simulink model "Simulink_TEP"  (R2024a)
settings: Solver=FixedStepAuto  StartTime=0.0  StopTime=5  FixedStep=1/3600  RelTol=1e-3
model workspace (MAT data in the model file):
  AD : Simulink.Parameter (value not decoded)
  AG : Simulink.Parameter (value not decoded)
  AH : Simulink.Parameter (value not decoded)
  AV : Simulink.Parameter (value not decoded)
  AVP : Simulink.Parameter (value not decoded)
  BCHL : Simulink.Parameter (value not decoded)
  BCHV : Simulink.Parameter (value not decoded)
  BD : Simulink.Parameter (value not decoded)
  BG : Simulink.Parameter (value not decoded)
  BH : Simulink.Parameter (value not decoded)
  BVP : Simulink.Parameter (value not decoded)
  CD : Simulink.Parameter (value not decoded)
  CG : Simulink.Parameter (value not decoded)
  CH : Simulink.Parameter (value not decoded)
  CVP : Simulink.Parameter (value not decoded)
  XMW : Simulink.Parameter (value not decoded)
symbols that are objects in the model workspace (value not decoded): AD, AG, AH, AV, AVP, BD, BG, BH, BVP, CD, CG, CH, CVP, XMW
undefined symbols (not defined in the file or in its folder): magnitude, SETPT, XMEAS, XMV
libraries: mylib x165, dspindex x17
(part 2 of 10)

== system Simulink_TEP/D Feed Stream 4/HST(4) Molar Enthalpy of Stream 4 MBtu//lb-mol ==
  TST(4) : Inport
  XST(I,4) : Inport  Port=2
  "Enthalpy of Stream " : mylib/Enthalpy of Stream   SystemSampleTime=-1  VariantActivationTime=update diagram  AllowFlexibleInterface=on  Latency=0  AutoFrameSizeCalculation=off
  ITY : Constant
  HST(4) : Outport  VectorParamsAs1DForOutWhenUnconnected=off
  wires:
  ITY/1 -> "Enthalpy of Stream "/1
  TST(4)/1 -> "Enthalpy of Stream "/2
  XST(I,4)/1 -> "Enthalpy of Stream "/3
  "Enthalpy of Stream "/1 -> HST(4)/1

== system Simulink_TEP/D Feed Stream 4/XST(I;4) Composition of Stream 4  ==
  TESUB8(1) : Inport
  TESUB8(2) : Inport  Port=2
  IDV(1) : Inport  Port=3
  IDV(2) : Inport  Port=4
  Bus Creator : BusCreator  Inputs=4
  Bus to Vector : BusToVector
  Constant : Constant  Value=0.03
  Constant1 : Constant  Value=2.43719e-3
  Constant2 : Constant  Value=0.005
  Constant3 : Constant
  Constant4 : Constant  Value=[XST4_D;XST4_E;XST4_F;XST4_G;XST4_H]
  Product : Product
  Product1 : Product
  Product2 : Product
  XST(1,4) : Sum  Inputs=+--
  XST(2,4) : Sum
  XST(3,4) : Sum  Inputs=+--
  XST(I;4) : Outport  PortDimensions=8  VectorParamsAs1DForOutWhenUnconnected=off
  wires:
  TESUB8(1)/1 -> XST(1,4)/1
  XST(1,4)/1 -> Bus Creator/1, XST(3,4)/2
  Product1/1 -> XST(1,4)/3
  IDV(1)/1 -> Product/1
  Constant3/1 -> XST(3,4)/1
  Product/1 -> XST(1,4)/2
  XST(2,4)/1 -> Bus Creator/2, XST(3,4)/3
  IDV(2)/1 -> Product2/1, Product1/1
  Constant2/1 -> Product2/2
  Constant/1 -> Product/2
  Constant1/1 -> Product1/2
  TESUB8(2)/1 -> XST(2,4)/1
  Product2/1 -> XST(2,4)/2
  XST(3,4)/1 -> Bus Creator/3
  Constant4/1 -> Bus Creator/4
  Bus Creator/1 -> Bus to Vector/1
  Bus to Vector/1 -> XST(I;4)/1

== system Simulink_TEP/Disturbances/Subsystem1 ==
  IDVWLK(2) : Inport
  Bus Creator : BusCreator  Inputs=6
  Bus Selector : BusSelector  OutputSignals=ADIST,BDIST,CDIST,DDIST,TNEXT,TLAST
  Delay{,1..5} (6 alike) : Delay  DelayLength=1  InitialCondition=0
  Subsystem2 : Subsystem
  TESUB8 : mylib/TESUB8  SystemSampleTime=-1  VariantActivationTime=update diagram  AllowFlexibleInterface=on  Latency=0  AutoFrameSizeCalculation=off
  TESUB8(2,Time) : Outport  PortDimensions=1  VectorParamsAs1DForOutWhenUnconnected=off
  tag scope: DIST2=global
  wires:
  TESUB8/1 -> TESUB8(2,Time)/1
  Bus Selector/6 -> Delay5/1  "<TLAST>"
  Bus Selector/5 -> Delay4/1  "<TNEXT>"
  Delay1/1 -> Bus Creator/2  "BDIST"
  Delay4/1 -> Bus Creator/5  "TNEXT"
  Delay5/1 -> Bus Creator/6  "TLAST"
  Subsystem2/1(DIST_NEW) -> TESUB8/1, Bus Selector/1
  IDVWLK(2)/1 -> Subsystem2/1(IDVWLK)
  Delay3/1 -> Bus Creator/4  "DDIST"
  Bus Selector/3 -> Delay2/1  "<CDIST>"
  Bus Selector/2 -> Delay1/1  "<BDIST>"
  Bus Creator/1 -> [DIST2], Subsystem2/2(DIST)
  Bus Selector/1 -> Delay/1  "<ADIST>"
  Delay2/1 -> Bus Creator/3  "CDIST"
  Bus Selector/4 -> Delay3/1  "<DDIST>"
  Delay/1 -> Bus Creator/1  "ADIST"

== system Simulink_TEP/Disturbances/Subsystem10 ==
  IDVWLK(10) : Inport
  Bus Creator : BusCreator  Inputs=6
  Bus Selector : BusSelector  OutputSignals=ADIST,BDIST,CDIST,DDIST,TNEXT,TLAST
  Delay{,1..6} (7 alike) : Delay  DelayLength=1  InitialCondition=0
  Subsystem3 : Subsystem
  TESUB8 : mylib/TESUB8  SystemSampleTime=-1  VariantActivationTime=update diagram  AllowFlexibleInterface=on  Latency=0  AutoFrameSizeCalculation=off
  TESUB8(10,Time) : Outport  VectorParamsAs1DForOutWhenUnconnected=off
  tag scope: DIST10=global, SWLK_10=global
  wires:
  TESUB8/1 -> TESUB8(10,Time)/1
  Delay/1 -> Bus Creator/1  "ADIST"
  Delay5/1 -> Bus Creator/6  "TLAST"
  Bus Selector/3 -> Delay2/1  "<CDIST>"
  Bus Selector/6 -> Delay5/1  "<TLAST>"
  Delay2/1 -> Bus Creator/3  "CDIST"
  Bus Selector/2 -> Delay1/1  "<BDIST>"
  Bus Creator/1 -> [DIST10], Subsystem3/2(DIST)
  Delay3/1 -> Bus Creator/4  "DDIST"
  Bus Selector/5 -> Delay4/1  "<TNEXT>"
  Delay4/1 -> Bus Creator/5  "TNEXT"
  Delay1/1 -> Bus Creator/2  "BDIST"
  Subsystem3/1(DIST_NEW) -> Bus Selector/1, TESUB8/1
  Bus Selector/4 -> Delay3/1  "<DDIST>"
  IDVWLK(10)/1 -> Subsystem3/1(IDVWLK)
  Bus Selector/1 -> Delay/1  "<ADIST>"
  Subsystem3/2(SWLK) -> Delay6/1
  Delay6/1 -> [SWLK_10]

== system Simulink_TEP/Disturbances/Subsystem11 ==
  IDVWLK(11) : Inport
  Bus Creator : BusCreator  Inputs=6
  Bus Selector : BusSelector  OutputSignals=ADIST,BDIST,CDIST,DDIST,TNEXT,TLAST
  Delay{,1..6} (7 alike) : Delay  DelayLength=1  InitialCondition=0
  Subsystem3 : Subsystem
  TESUB8 : mylib/TESUB8  SystemSampleTime=-1  VariantActivationTime=update diagram  AllowFlexibleInterface=on  Latency=0  AutoFrameSizeCalculation=off
  TESUB8(11,Time) : Outport  VectorParamsAs1DForOutWhenUnconnected=off
  tag scope: DIST11=global, SWLK_11=global
  wires:
  TESUB8/1 -> TESUB8(11,Time)/1
  Delay6/1 -> [SWLK_11]
  IDVWLK(11)/1 -> Subsystem3/1(IDVWLK)
  Bus Selector/1 -> Delay/1  "<ADIST>"
  Bus Selector/4 -> Delay3/1  "<DDIST>"
  Subsystem3/1(DIST_NEW) -> TESUB8/1, Bus Selector/1
  Bus Selector/5 -> Delay4/1  "<TNEXT>"
  Delay3/1 -> Bus Creator/4  "DDIST"
  Delay4/1 -> Bus Creator/5  "TNEXT"
  Delay1/1 -> Bus Creator/2  "BDIST"
  Bus Selector/2 -> Delay1/1  "<BDIST>"
  Delay2/1 -> Bus Creator/3  "CDIST"
  Bus Selector/6 -> Delay5/1  "<TLAST>"
  Delay/1 -> Bus Creator/1  "ADIST"
  Delay5/1 -> Bus Creator/6  "TLAST"
  Bus Creator/1 -> [DIST11], Subsystem3/2(DIST)
  Subsystem3/2(SWLK) -> Delay6/1
  Bus Selector/3 -> Delay2/1  "<CDIST>"

== system Simulink_TEP/Disturbances/Subsystem12 ==
  IDVWLK(12) : Inport
  Bus Creator : BusCreator  Inputs=6
  Bus Selector : BusSelector  OutputSignals=ADIST,BDIST,CDIST,DDIST,TNEXT,TLAST
  Delay{,1..6} (7 alike) : Delay  DelayLength=1  InitialCondition=0
  Subsystem3 : Subsystem
  TESUB8 : mylib/TESUB8  SystemSampleTime=-1  VariantActivationTime=update diagram  AllowFlexibleInterface=on  Latency=0  AutoFrameSizeCalculation=off
  TESUB8(12,Time) : Outport  VectorParamsAs1DForOutWhenUnconnected=off
  tag scope: DIST12=global, SWLK_12=global
  wires:
  TESUB8/1 -> TESUB8(12,Time)/1
  Delay6/1 -> [SWLK_12]
  IDVWLK(12)/1 -> Subsystem3/1(IDVWLK)
  Bus Selector/1 -> Delay/1  "<ADIST>"
  Bus Selector/4 -> Delay3/1  "<DDIST>"
  Subsystem3/1(DIST_NEW) -> TESUB8/1, Bus Selector/1
  Bus Selector/5 -> Delay4/1  "<TNEXT>"
  Delay3/1 -> Bus Creator/4  "DDIST"
  Delay4/1 -> Bus Creator/5  "TNEXT"
  Delay1/1 -> Bus Creator/2  "BDIST"
  Bus Selector/2 -> Delay1/1  "<BDIST>"
  Delay2/1 -> Bus Creator/3  "CDIST"
  Bus Selector/6 -> Delay5/1  "<TLAST>"
  Delay/1 -> Bus Creator/1  "ADIST"
  Delay5/1 -> Bus Creator/6  "TLAST"
  Bus Creator/1 -> [DIST12], Subsystem3/2(DIST)
  Subsystem3/2(SWLK) -> Delay6/1
  Bus Selector/3 -> Delay2/1  "<CDIST>"

== system Simulink_TEP/Disturbances/Subsystem2 ==
  IDVWLK(1) : Inport
  Bus Creator : BusCreator  Inputs=6
  Bus Selector : BusSelector  OutputSignals=ADIST,BDIST,CDIST,DDIST,TNEXT,TLAST
  Delay{,1..5} (6 alike) : Delay  DelayLength=1  InitialCondition=0
  Subsystem : Subsystem
  TESUB8 : mylib/TESUB8  SystemSampleTime=-1  VariantActivationTime=update diagram  AllowFlexibleInterface=on  Latency=0  AutoFrameSizeCalculation=off
  TESUB8(1,Time) : Outport  VectorParamsAs1DForOutWhenUnconnected=off
  tag scope: DIST1=global
  wires:
  TESUB8/1 -> TESUB8(1,Time)/1
  Subsystem/1(DIST_NEW) -> TESUB8/1, Bus Selector/1
  IDVWLK(1)/1 -> Subsystem/1(IDVWLK)
  Bus Creator/1 -> [DIST1], Subsystem/2(DIST)
  Bus Selector/1 -> Delay/1  "<ADIST>"
  Delay/1 -> Bus Creator/1  "ADIST"
  Bus Selector/2 -> Delay1/1  "<BDIST>"
  Delay1/1 -> Bus Creator/2  "BDIST"
  Bus Selector/3 -> Delay2/1  "<CDIST>"
  Delay2/1 -> Bus Creator/3  "CDIST"
  Delay3/1 -> Bus Creator/4  "DDIST"
  Bus Selector/4 -> Delay3/1  "<DDIST>"
  Delay4/1 -> Bus Creator/5  "TNEXT"
  Bus Selector/5 -> Delay4/1  "<TNEXT>"
  Delay5/1 -> Bus Creator/6  "TLAST"
  Bus Selector/6 -> Delay5/1  "<TLAST>"

== system Simulink_TEP/Disturbances/Subsystem3 ==
  IDVWLK(3) : Inport
  Bus Creator : BusCreator  Inputs=6
  Bus Selector : BusSelector  OutputSignals=ADIST,BDIST,CDIST,DDIST,TNEXT,TLAST
  Delay{,1..5} (6 alike) : Delay  DelayLength=1  InitialCondition=0
  Subsystem2 : Subsystem
  TESUB8 : mylib/TESUB8  SystemSampleTime=-1  VariantActivationTime=update diagram  AllowFlexibleInterface=on  Latency=0  AutoFrameSizeCalculation=off
  TESUB8(3,Time) : Outport  PortDimensions=1  VectorParamsAs1DForOutWhenUnconnected=off
  tag scope: DIST3=global
  wires:
  TESUB8/1 -> TESUB8(3,Time)/1
  IDVWLK(3)/1 -> Subsystem2/1(IDVWLK)
  Bus Selector/1 -> Delay/1  "<ADIST>"
  Delay/1 -> Bus Creator/1  "ADIST"
  Delay2/1 -> Bus Creator/3  "CDIST"
  Subsystem2/1(DIST_NEW) -> TESUB8/1, Bus Selector/1
  Delay5/1 -> Bus Creator/6  "TLAST"
  Delay4/1 -> Bus Creator/5  "TNEXT"
  Delay3/1 -> Bus Creator/4  "DDIST"
  Bus Selector/6 -> Delay5/1  "<TLAST>"
  Bus Creator/1 -> [DIST3], Subsystem2/2(DIST)
  Bus Selector/4 -> Delay3/1  "<DDIST>"
  Delay1/1 -> Bus Creator/2  "BDIST"
  Bus Selector/2 -> Delay1/1  "<BDIST>"
  Bus Selector/3 -> Delay2/1  "<CDIST>"
  Bus Selector/5 -> Delay4/1  "<TNEXT>"

== system Simulink_TEP/Disturbances/Subsystem4 ==
  IDVWLK(4) : Inport
  Bus Creator : BusCreator  Inputs=6
  Bus Selector : BusSelector  OutputSignals=ADIST,BDIST,CDIST,DDIST,TNEXT,TLAST
  Delay{,1..5} (6 alike) : Delay  DelayLength=1  InitialCondition=0
  Subsystem2 : Subsystem
  TESUB8 : mylib/TESUB8  SystemSampleTime=-1  VariantActivationTime=update diagram  AllowFlexibleInterface=on  Latency=0  AutoFrameSizeCalculation=off
  TESUB8(4,Time) : Outport  PortDimensions=1  VectorParamsAs1DForOutWhenUnconnected=off
  tag scope: DIST4=global
  wires:
  TESUB8/1 -> TESUB8(4,Time)/1
  Subsystem2/1(DIST_NEW) -> TESUB8/1, Bus Selector/1
  Bus Selector/6 -> Delay5/1  "<TLAST>"
  Bus Selector/5 -> Delay4/1  "<TNEXT>"
  Delay1/1 -> Bus Creator/2  "BDIST"
  Delay4/1 -> Bus Creator/5  "TNEXT"
  Delay5/1 -> Bus Creator/6  "TLAST"
  IDVWLK(4)/1 -> Subsystem2/1(IDVWLK)
  Delay3/1 -> Bus Creator/4  "DDIST"
  Bus Selector/3 -> Delay2/1  "<CDIST>"
  Bus Selector/2 -> Delay1/1  "<BDIST>"
  Bus Creator/1 -> [DIST4], Subsystem2/2(DIST)
  Bus Selector/1 -> Delay/1  "<ADIST>"
  Delay2/1 -> Bus Creator/3  "CDIST"
  Bus Selector/4 -> Delay3/1  "<DDIST>"
  Delay/1 -> Bus Creator/1  "ADIST"

== system Simulink_TEP/Disturbances/Subsystem5 ==
  IDVWLK(5) : Inport
  Bus Creator : BusCreator  Inputs=6
  Bus Selector : BusSelector  OutputSignals=ADIST,BDIST,CDIST,DDIST,TNEXT,TLAST
  Delay{,1..5} (6 alike) : Delay  DelayLength=1  InitialCondition=0
  Subsystem2 : Subsystem
  TESUB8 : mylib/TESUB8  SystemSampleTime=-1  VariantActivationTime=update diagram  AllowFlexibleInterface=on  Latency=0  AutoFrameSizeCalculation=off
  TESUB8(5,Time) : Outport  PortDimensions=1  VectorParamsAs1DForOutWhenUnconnected=off
  tag scope: DIST5=global
  wires:
  TESUB8/1 -> TESUB8(5,Time)/1
  Bus Selector/6 -> Delay5/1  "<TLAST>"
  Bus Selector/5 -> Delay4/1  "<TNEXT>"
  Delay1/1 -> Bus Creator/2  "BDIST"
  Delay4/1 -> Bus Creator/5  "TNEXT"
  Delay5/1 -> Bus Creator/6  "TLAST"
  Subsystem2/1(DIST_NEW) -> TESUB8/1, Bus Selector/1
  IDVWLK(5)/1 -> Subsystem2/1(IDVWLK)
  Delay3/1 -> Bus Creator/4  "DDIST"
  Bus Selector/3 -> Delay2/1  "<CDIST>"
  Bus Selector/2 -> Delay1/1  "<BDIST>"
  Bus Creator/1 -> [DIST5], Subsystem2/2(DIST)
  Bus Selector/1 -> Delay/1  "<ADIST>"
  Delay2/1 -> Bus Creator/3  "CDIST"
  Bus Selector/4 -> Delay3/1  "<DDIST>"
  Delay/1 -> Bus Creator/1  "ADIST"

== system Simulink_TEP/Disturbances/Subsystem6 ==
  IDVWLK(6) : Inport
  Bus Creator : BusCreator  Inputs=6
  Bus Selector : BusSelector  OutputSignals=ADIST,BDIST,CDIST,DDIST,TNEXT,TLAST
  Delay{,1..5} (6 alike) : Delay  DelayLength=1  InitialCondition=0
  Subsystem2 : Subsystem
  TESUB8 : mylib/TESUB8  SystemSampleTime=-1  VariantActivationTime=update diagram  AllowFlexibleInterface=on  Latency=0  AutoFrameSizeCalculation=off
  TESUB8(6,Time) : Outport  PortDimensions=1  VectorParamsAs1DForOutWhenUnconnected=off
  tag scope: DIST6=global
  wires:
  TESUB8/1 -> TESUB8(6,Time)/1
  Bus Selector/6 -> Delay5/1  "<TLAST>"
  Bus Selector/5 -> Delay4/1  "<TNEXT>"
  Delay1/1 -> Bus Creator/2  "BDIST"
  Delay4/1 -> Bus Creator/5  "TNEXT"
  Delay5/1 -> Bus Creator/6  "TLAST"
  Subsystem2/1(DIST_NEW) -> TESUB8/1, Bus Selector/1
  IDVWLK(6)/1 -> Subsystem2/1(IDVWLK)
  Delay3/1 -> Bus Creator/4  "DDIST"
  Bus Selector/3 -> Delay2/1  "<CDIST>"
  Bus Selector/2 -> Delay1/1  "<BDIST>"
  Bus Creator/1 -> [DIST6], Subsystem2/2(DIST)
  Bus Selector/1 -> Delay/1  "<ADIST>"
  Delay2/1 -> Bus Creator/3  "CDIST"
  Bus Selector/4 -> Delay3/1  "<DDIST>"
  Delay/1 -> Bus Creator/1  "ADIST"

== system Simulink_TEP/Disturbances/Subsystem7 ==
  IDVWLK(7) : Inport
  Bus Creator : BusCreator  Inputs=6
  Bus Selector : BusSelector  OutputSignals=ADIST,BDIST,CDIST,DDIST,TNEXT,TLAST
  Delay{,1..5} (6 alike) : Delay  DelayLength=1  InitialCondition=0
  Subsystem2 : Subsystem
  TESUB8 : mylib/TESUB8  SystemSampleTime=-1  VariantActivationTime=update diagram  AllowFlexibleInterface=on  Latency=0  AutoFrameSizeCalculation=off
  TESUB8(7,Time) : Outport  PortDimensions=1  VectorParamsAs1DForOutWhenUnconnected=off
  tag scope: DIST7=global
  wires:
  TESUB8/1 -> TESUB8(7,Time)/1
  Bus Selector/6 -> Delay5/1  "<TLAST>"
  Bus Selector/5 -> Delay4/1  "<TNEXT>"
  Delay1/1 -> Bus Creator/2  "BDIST"
  Delay4/1 -> Bus Creator/5  "TNEXT"
  Delay5/1 -> Bus Creator/6  "TLAST"
  Subsystem2/1(DIST_NEW) -> TESUB8/1, Bus Selector/1
  IDVWLK(7)/1 -> Subsystem2/1(IDVWLK)
  Delay3/1 -> Bus Creator/4  "DDIST"
  Bus Selector/3 -> Delay2/1  "<CDIST>"
  Bus Selector/2 -> Delay1/1  "<BDIST>"
  Bus Creator/1 -> [DIST7], Subsystem2/2(DIST)
  Bus Selector/1 -> Delay/1  "<ADIST>"
  Delay2/1 -> Bus Creator/3  "CDIST"
  Bus Selector/4 -> Delay3/1  "<DDIST>"
  Delay/1 -> Bus Creator/1  "ADIST"

== system Simulink_TEP/Disturbances/Subsystem8 ==
  IDVWLK(8) : Inport
  Bus Creator : BusCreator  Inputs=6
  Bus Selector : BusSelector  OutputSignals=ADIST,BDIST,CDIST,DDIST,TNEXT,TLAST
  Delay{,1..5} (6 alike) : Delay  DelayLength=1  InitialCondition=0
  Subsystem2 : Subsystem
  TESUB8 : mylib/TESUB8  SystemSampleTime=-1  VariantActivationTime=update diagram  AllowFlexibleInterface=on  Latency=0  AutoFrameSizeCalculation=off
  TESUB8(8,Time) : Outport  PortDimensions=1  VectorParamsAs1DForOutWhenUnconnected=off
  tag scope: DIST8=global
  wires:
  TESUB8/1 -> TESUB8(8,Time)/1
  Bus Selector/6 -> Delay5/1  "<TLAST>"
  Bus Selector/5 -> Delay4/1  "<TNEXT>"
  Delay1/1 -> Bus Creator/2  "BDIST"
  Delay4/1 -> Bus Creator/5  "TNEXT"
  Delay5/1 -> Bus Creator/6  "TLAST"
  Subsystem2/1(DIST_NEW) -> TESUB8/1, Bus Selector/1
  IDVWLK(8)/1 -> Subsystem2/1(IDVWLK)
  Delay3/1 -> Bus Creator/4  "DDIST"
  Bus Selector/3 -> Delay2/1  "<CDIST>"
  Bus Selector/2 -> Delay1/1  "<BDIST>"
  Bus Creator/1 -> [DIST8], Subsystem2/2(DIST)
  Bus Selector/1 -> Delay/1  "<ADIST>"
  Delay2/1 -> Bus Creator/3  "CDIST"
  Bus Selector/4 -> Delay3/1  "<DDIST>"
  Delay/1 -> Bus Creator/1  "ADIST"

== system Simulink_TEP/Disturbances/Subsystem9 ==
  IDVWLK(9) : Inport
  Bus Creator : BusCreator  Inputs=6
  Bus Selector : BusSelector  OutputSignals=ADIST,BDIST,CDIST,DDIST,TNEXT,TLAST
  Delay{,1..5} (6 alike) : Delay  DelayLength=1  InitialCondition=0
  Subsystem2 : Subsystem
  TESUB8 : mylib/TESUB8  SystemSampleTime=-1  VariantActivationTime=update diagram  AllowFlexibleInterface=on  Latency=0  AutoFrameSizeCalculation=off
  TESUB8(9,Time) : Outport  VectorParamsAs1DForOutWhenUnconnected=off
  tag scope: DIST9=global
  wires:
  TESUB8/1 -> TESUB8(9,Time)/1
  Bus Selector/6 -> Delay5/1  "<TLAST>"
  Bus Selector/5 -> Delay4/1  "<TNEXT>"
  Delay1/1 -> Bus Creator/2  "BDIST"
  Delay4/1 -> Bus Creator/5  "TNEXT"
  Delay5/1 -> Bus Creator/6  "TLAST"
  Subsystem2/1(DIST_NEW) -> TESUB8/1, Bus Selector/1
  IDVWLK(9)/1 -> Subsystem2/1(IDVWLK)
  Delay3/1 -> Bus Creator/4  "DDIST"
  Bus Selector/3 -> Delay2/1  "<CDIST>"
  Bus Selector/2 -> Delay1/1  "<BDIST>"
  Bus Creator/1 -> [DIST9], Subsystem2/2(DIST)
  Bus Selector/1 -> Delay/1  "<ADIST>"
  Delay2/1 -> Bus Creator/3  "CDIST"
  Bus Selector/4 -> Delay3/1  "<DDIST>"
  Delay/1 -> Bus Creator/1  "ADIST"

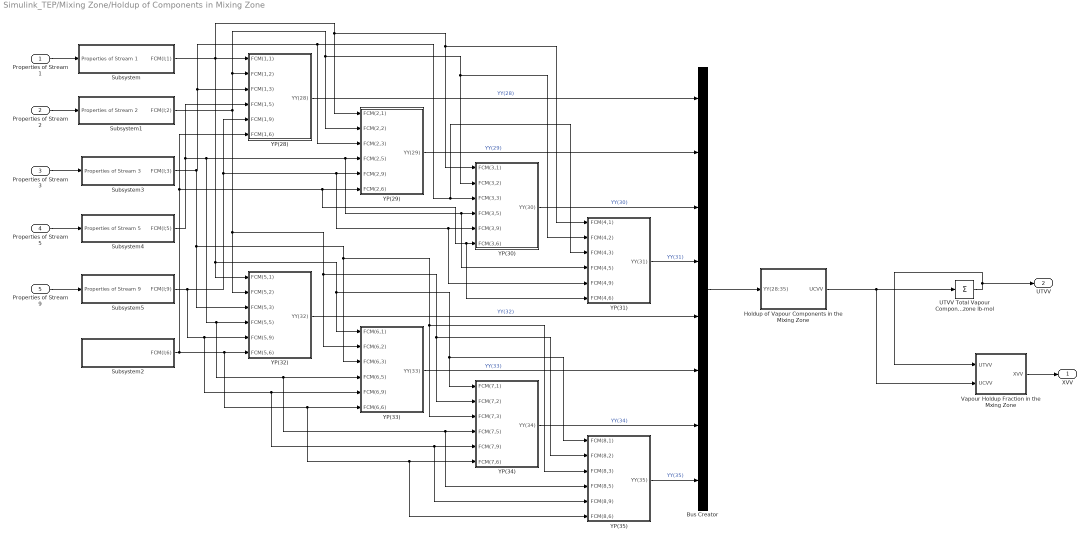
== system Simulink_TEP/Mixing Zone/Holdup of Components in Mixing Zone ==
  Properties of Stream 1 : Inport
  Properties of Stream 2 : Inport  Port=2
  Properties of Stream 3 : Inport  Port=3
  Properties of Stream 5 : Inport  Port=4
  Properties of Stream 9 : Inport  Port=5
  Bus Creator : BusCreator  Inputs=8
  Holdup of Vapour Components in the Mixing Zone : Subsystem
  Subsystem : Subsystem
  Subsystem1 : Subsystem
  Subsystem2 : Subsystem
  Subsystem3 : Subsystem
  Subsystem4 : Subsystem
  Subsystem5 : Subsystem
  UTVV Total Vapour Component holdup in Mixing zone lb-mol : Sum  Inputs=+
  Vapour Holdup Fraction in the Mxing Zone : Subsystem
  YP(28) : Subsystem
  YP(29) : Subsystem
  YP(30) : Subsystem
  YP(31) : Subsystem
  YP(32) : Subsystem
  YP(33) : Subsystem
  YP(34) : Subsystem
  YP(35) : Subsystem
  XVV : Outport  PortDimensions=8  VectorParamsAs1DForOutWhenUnconnected=off
  UTVV : Outport  Port=2  PortDimensions=1  VectorParamsAs1DForOutWhenUnconnected=off
  wires:
  YP(28)/1(YY(28)) -> Bus Creator/1  "YY(28)"
  YP(29)/1(YY(29)) -> Bus Creator/2  "YY(29)"
  YP(30)/1(YY(30)) -> Bus Creator/3  "YY(30)"
  YP(31)/1(YY(31)) -> Bus Creator/4  "YY(31)"
  YP(32)/1(YY(32)) -> Bus Creator/5  "YY(32)"
  YP(33)/1(YY(33)) -> Bus Creator/6  "YY(33)"
  YP(34)/1(YY(34)) -> Bus Creator/7  "YY(34)"
  YP(35)/1(YY(35)) -> Bus Creator/8  "YY(35)"
  Bus Creator/1 -> Holdup of Vapour Components in the Mixing Zone/1(YY(28:35))
  Holdup of Vapour Components in the Mixing Zone/1(UCVV) -> Vapour Holdup Fraction in the Mxing Zone/2(UCVV), UTVV Total Vapour Component holdup in Mixing zone lb-mol/1
  UTVV Total Vapour Component holdup in Mixing zone lb-mol/1 -> UTVV/1, Vapour Holdup Fraction in the Mxing Zone/1(UTVV)
  Vapour Holdup Fraction in the Mxing Zone/1(XVV) -> XVV/1
  Properties of Stream 1/1 -> Subsystem/1(Properties of Stream 1)
  Properties of Stream 2/1 -> Subsystem1/1(Properties of Stream 2)
  Properties of Stream 3/1 -> Subsystem3/1(Properties of Stream 3)
  Properties of Stream 5/1 -> Subsystem4/1(Properties of Stream 5)
  Properties of Stream 9/1 -> Subsystem5/1(Properties of Stream 9)
  Subsystem/1(FCM(I;1)) -> YP(35)/1(FCM(8,1)), YP(34)/1(FCM(7,1)), YP(33)/1(FCM(6,1)), YP(32)/1(FCM(5,1)), YP(31)/1(FCM(4,1)), YP(30)/1(FCM(3,1)), YP(29)/1(FCM(2,1)), YP(28)/1(FCM(1,1))
  Subsystem1/1(FCM(I;2)) -> YP(35)/2(FCM(8,2)), YP(34)/2(FCM(7,2)), YP(33)/2(FCM(6,2)), YP(32)/2(FCM(5,2)), YP(31)/2(FCM(4,2)), YP(30)/2(FCM(3,2)), YP(29)/2(FCM(2,2)), YP(28)/2(FCM(1,2))
  Subsystem3/1(FCM(I;3)) -> YP(35)/3(FCM(8,3)), YP(34)/3(FCM(7,3)), YP(33)/3(FCM(6,3)), YP(32)/3(FCM(5,3)), YP(29)/3(FCM(2,3)), YP(31)/3(FCM(4,3)), YP(30)/3(FCM(3,3)), YP(28)/3(FCM(1,3))
  Subsystem4/1(FCM(I;5)) -> YP(35)/4(FCM(8,5)), YP(34)/4(FCM(7,5)), YP(33)/4(FCM(6,5)), YP(32)/4(FCM(5,5)), YP(31)/4(FCM(4,5)), YP(30)/4(FCM(3,5)), YP(29)/4(FCM(2,5)), YP(28)/4(FCM(1,5))
  Subsystem5/1(FCM(I;9)) -> YP(35)/5(FCM(8,9)), YP(34)/5(FCM(7,9)), YP(33)/5(FCM(6,9)), YP(32)/5(FCM(5,9)), YP(31)/5(FCM(4,9)), YP(30)/5(FCM(3,9)), YP(29)/5(FCM(2,9)), YP(28)/5(FCM(1,9))
  Subsystem2/1(FCM(I;6)) -> YP(35)/6(FCM(8,6)), YP(34)/6(FCM(7,6)), YP(33)/6(FCM(6,6)), YP(32)/6(FCM(5,6)), YP(31)/6(FCM(4,6)), YP(30)/6(FCM(3,6)), YP(29)/6(FCM(2,6)), YP(28)/6(FCM(1,6))

== system Simulink_TEP/Mixing Zone/Internal energy of mixing zone ==
  Properties of Stream 1 : Inport
  Properties of Stream 2 : Inport  Port=2
  Properties of Stream 3 : Inport  Port=3
  Properties of Stream 5 : Inport  Port=4
  Properties of Stream 9 : Inport  Port=5
  Add : Sum  Inputs=+++++-
  Bus Selector : BusSelector  OutputSignals=HST(1),FTM(1)
  Bus Selector1 : BusSelector  OutputSignals=HST(2),FTM(2)
  Bus Selector2 : BusSelector  OutputSignals=HST(3),FTM(3)
  Bus Selector3 : BusSelector  OutputSignals=HST(5),FTM(5)
  Bus Selector4 : BusSelector  OutputSignals=HST(9),FTM(9)
  Bus Selector5 : BusSelector  OutputSignals=signal1.HST(6) = HST(7),signal1.FTM(6) = FTM(7)
  Product{,1..5} (6 alike) : Product
  YP(36) : Integrator  InitialConditionSource=external
  YY(36) : Constant  Value=0.9218489762
  "YY(36) " : Outport  VectorParamsAs1DForOutWhenUnconnected=off
  wires:
  Bus Selector/1 -> Product/1  "<HST(1)>"
  Bus Selector/2 -> Product/2  "<FTM(1)>"
  Bus Selector1/2 -> Product1/2  "<FTM(2)>"
  Bus Selector1/1 -> Product1/1  "<HST(2)>"
  Product/1 -> Add/1
  Product1/1 -> Add/2
  YP(36)/1 -> "YY(36) "/1
  YY(36)/1 -> YP(36)/2
  Add/1 -> YP(36)/1
  Bus Selector3/1 -> Product3/1  "<HST(5)>"
  Bus Selector2/2 -> Product2/2  "<FTM(3)>"
  Product2/1 -> Add/3
  Bus Selector3/2 -> Product3/2  "<FTM(5)>"
  Product3/1 -> Add/4
  Bus Selector2/1 -> Product2/1  "<HST(3)>"
  Bus Selector4/2 -> Product4/2  "<FTM(9)>"
  Bus Selector5/1 -> Product5/1  "<HST(6) = HST(7)>"
  Bus Selector4/1 -> Product4/1  "<HST(9)>"
  Product5/1 -> Add/6
  Product4/1 -> Add/5
  Bus Selector5/2 -> Product5/2  "<FTM(6) = FTM(7)>"
  Properties of Stream 1/1 -> Bus Selector/1
  Properties of Stream 2/1 -> Bus Selector1/1
  Properties of Stream 3/1 -> Bus Selector2/1
  Properties of Stream 5/1 -> Bus Selector3/1
  Properties of Stream 9/1 -> Bus Selector4/1
  [PropertiesStream6] -> Bus Selector5/1

== system Simulink_TEP/Mixing Zone/PTV Total pressure of Mixing zone mmHg ==
  UTVV : Inport
  TCV : Inport  Port=2
  PTV Total pressure of Mixing zone mmHg : Product  Inputs=***/
  RG Universal Gas Constant ft³·mmHg/K·lb-mol : Constant  Value=998.9
  TKV Temperature in Mixing zone K : Sum
  To Convert °C to K : Constant  Value=273.15
  VTV Total Volume of Mixing zone ft³ : Constant  Value=5000
  PTV : Outport  VectorParamsAs1DForOutWhenUnconnected=off
  wires:
  RG Universal Gas Constant ft³·mmHg/K·lb-mol/1 -> PTV Total pressure of Mixing zone mmHg/2
  VTV Total Volume of Mixing zone ft³/1 -> PTV Total pressure of Mixing zone mmHg/4
  TKV Temperature in Mixing zone K/1 -> PTV Total pressure of Mixing zone mmHg/3
  TCV/1 -> TKV Temperature in Mixing zone K/1
  PTV Total pressure of Mixing zone mmHg/1 -> PTV/1
  To Convert °C to K/1 -> TKV Temperature in Mixing zone K/2
  UTVV/1 -> PTV Total pressure of Mixing zone mmHg/1

== system Simulink_TEP/Mixing Zone/Stream 6 ==
  XST(I,6) : Inport
  TST(6) : Inport  Port=2  PortDimensions=1
  Bus Creator : BusCreator  Inputs=6
  FCM(I,6) Component molar flow of Stream 6 lb-mol/h : Product
  FTM(6) : Product  Inputs=*/
  HST(6) Molar Enthalpy of Stream 6 MBtu/lb-mol : Subsystem
  ITY : Constant
  Subsystem : Subsystem
  XMWS(6) Molecular weight of Stream 6 lb/lb-mol : Subsystem
  Properties of Stream 6 : Outport  VectorParamsAs1DForOutWhenUnconnected=off
  wires:
  XMWS(6) Molecular weight of Stream 6 lb/lb-mol/1(XMWS(6)) -> FTM(6)/2
  ITY/1 -> Bus Creator/6, HST(6) Molar Enthalpy of Stream 6 MBtu/lb-mol/1(ITY)  "Phase"
  XST(I,6)/1 -> Bus Creator/1, HST(6) Molar Enthalpy of Stream 6 MBtu/lb-mol/3(XST(I,6)), FCM(I,6) Component molar flow of Stream 6 lb-mol/h/1, XMWS(6) Molecular weight of Stream 6 lb/lb-mol/1(XST(I,6))  "XST(I;6) = XST(I;7)"
  TST(6)/1 -> Bus Creator/2, HST(6) Molar Enthalpy of Stream 6 MBtu/lb-mol/2(T)  "TST(6) = TST(7)"
  HST(6) Molar Enthalpy of Stream 6 MBtu/lb-mol/1("H ") -> Bus Creator/3  "HST(6) = HST(7)"
  FTM(6)/1 -> FCM(I,6) Component molar flow of Stream 6 lb-mol/h/2, Bus Creator/4  "FTM(6) = FTM(7)"
  FCM(I,6) Component molar flow of Stream 6 lb-mol/h/1 -> Bus Creator/5  "FCM(I;6) = FCM(I;7)"
  Bus Creator/1 -> Properties of Stream 6/1
  Subsystem/1("FLMS ") -> FTM(6)/1

== system Simulink_TEP/Mixing Zone/TCV Initial Temperature in Mixing zone °C  ==
  UTVV : Inport
  ETV : Inport  Port=2  PortDimensions=1
  XVV : Inport  Port=3
  "AG(I) Coefficient A to determine Enthalpy MBtu/lb·°F " : Constant  Value=AG
  "AH(I) Coefficient A to determine Enthalpy MBtu/lb·°F " : Constant  Value=AH
  AV(I) Coefficient AV to determine Enthalpy MBtu/lb : Constant  Value=AV
  BG(I) Coefficient B to determine Enthalpy MBtu/lb·°F² : Constant  Value=BG
  BH(I) Coefficient B to determine Enthalpy MBtu/lb·°F² : Constant  Value=BH
  CG(I) Coefficient C to determine Enthalpy MBtu/lb·°F³ : Constant  Value=CG
  CH(I) Coefficient C to determine Enthalpy MBtu/lb·°F³ : Constant  Value=CH
  Delay : Delay  DelayLength=1  InitialCondition=0
  Display1 : Display
  IC : InitialCondition  Value=0
  ITY : Constant  Value=2
  MATLAB Function : MATLAB Function  TreatAsAtomicUnit=on
  "XMW(I) Molecular weight of components lb/lb-mol " : Constant  Value=XMW
  TCV : Outport  PortDimensions=1  VectorParamsAs1DForOutWhenUnconnected=off
  wires:
  MATLAB Function/1(TCV) -> TCV/1, Delay/1
  IC/1 -> MATLAB Function/13("TCV ")
  "AG(I) Coefficient A to determine Enthalpy MBtu/lb·°F "/1 -> MATLAB Function/4(AG)
  AV(I) Coefficient AV to determine Enthalpy MBtu/lb/1 -> MATLAB Function/7(AV)
  MATLAB Function/2(J) -> Display1/1
  ETV/1 -> MATLAB Function/10(ETV)
  CH(I) Coefficient C to determine Enthalpy MBtu/lb·°F³/1 -> MATLAB Function/3(CH)
  UTVV/1 -> MATLAB Function/11(UTVV)
  ITY/1 -> MATLAB Function/12(ITY)
  "XMW(I) Molecular weight of components lb/lb-mol "/1 -> MATLAB Function/8(XMW)
  XVV/1 -> MATLAB Function/9(XVV)
  "AH(I) Coefficient A to determine Enthalpy MBtu/lb·°F "/1 -> MATLAB Function/1(AH)
  CG(I) Coefficient C to determine Enthalpy MBtu/lb·°F³/1 -> MATLAB Function/6(CG)
  BH(I) Coefficient B to determine Enthalpy MBtu/lb·°F²/1 -> MATLAB Function/2(BH)
  BG(I) Coefficient B to determine Enthalpy MBtu/lb·°F²/1 -> MATLAB Function/5(BG)
  Delay/1 -> IC/1

== system Simulink_TEP/Process Measurements/Compressor Work ==
  Add : Sum
  Bus Selector1 : BusSelector  OutputSignals=signal4.XMNS(20)
  XMEAS(20) : Gain  Gain=0.29307E3
  "XMEAS(20) " : Outport  VectorParamsAs1DForOutWhenUnconnected=off
  wires:
  [CPDH] -> XMEAS(20)/1
  XMEAS(20)/1 -> Add/1
  Add/1 -> "XMEAS(20) "/1  "XMEAS(20)"
  [XMNS] -> Bus Selector1/1
  Bus Selector1/1 -> Add/2  "<XMNS(20)>"

== system Simulink_TEP/Process Measurements/Condenser Cooling Outlet Water Temperature ==
  Add : Sum
  Bus Selector1 : BusSelector  OutputSignals=signal4.XMNS(22)
  XMEAS(22) : Outport  PortDimensions=1  VectorParamsAs1DForOutWhenUnconnected=off
  wires:
  [TWS] -> Add/1
  Add/1 -> XMEAS(22)/1  "XMEAS(22)"
  [XMNS] -> Bus Selector1/1
  Bus Selector1/1 -> Add/2  "<XMNS(22)>"

== system Simulink_TEP/Process Measurements/Feed Streams ==
  " A Feed" : Subsystem
  A and C Feed : Subsystem
  Bus Creator2 : BusCreator  Inputs=5
  D Feed : Subsystem
  E Feed : Subsystem
  Recycle Flow : Subsystem
  XMEASF : Outport  VectorParamsAs1DForOutWhenUnconnected=off
  wires:
  " A Feed"/1("XMEAS(1) ") -> Bus Creator2/1
  E Feed/1("XMEAS(3) ") -> Bus Creator2/3
  A and C Feed/1("XMEAS(4) ") -> Bus Creator2/4
  Bus Creator2/1 -> XMEASF/1
  D Feed/1("XMEAS(2) ") -> Bus Creator2/2
  Recycle Flow/1("XMEAS(5) ") -> Bus Creator2/5

== system Simulink_TEP/Process Measurements/Product analysis ==
  Bus Creator : BusCreator  Inputs=5
  Bus Selector : BusSelector  OutputSignals=XST(I;13)
  Scope : Scope
  Subsystem : Subsystem
  XMEAS : Outport  VectorParamsAs1DForOutWhenUnconnected=off
  wires:
  [PropertiesStream13] -> Bus Selector/1
  Bus Creator/1 -> Scope/1, XMEAS/1
  Bus Selector/1 -> Subsystem/1(<XST(I;13)>)  "<XST(I;13)>"
  Subsystem/1(XMEAS(37)) -> Bus Creator/1  "XMEAS(37)"
  Subsystem/2(XMEAS(38)) -> Bus Creator/2  "XMEAS(38)"
  Subsystem/3(XMEAS(39)) -> Bus Creator/3  "XMEAS(39)"
  Subsystem/4(XMEAS(40)) -> Bus Creator/4  "XMEAS(40)"
  Subsystem/5(XMEAS(41)) -> Bus Creator/5  "XMEAS(41)"

== system Simulink_TEP/Process Measurements/Purge gas analysis ==
  Bus Creator : BusCreator  Inputs=8
  Bus Selector : BusSelector  OutputSignals=signal1.XST(I;10)
  Subsystem : Subsystem
  XMEASP : Outport  VectorParamsAs1DForOutWhenUnconnected=off
  wires:
  [PropertiesStream10] -> Bus Selector/1
  Bus Creator/1 -> XMEASP/1
  Bus Selector/1 -> Subsystem/1(<XST(I;10)>)  "<XST(I;10)>"
  Subsystem/1(XMEAS(29)) -> Bus Creator/1  "XMEAS(29)"
  Subsystem/2(XMEAS(30)) -> Bus Creator/2  "XMEAS(30)"
  Subsystem/3(XMEAS(31)) -> Bus Creator/3  "XMEAS(31)"
  Subsystem/4(XMEAS(32)) -> Bus Creator/4  "XMEAS(32)"
  Subsystem/5(XMEAS(33)) -> Bus Creator/5  "XMEAS(33)"
  Subsystem/6(XMEAS(34)) -> Bus Creator/6  "XMEAS(34)"
  Subsystem/7(XMEAS(35)) -> Bus Creator/7  "XMEAS(35)"
  Subsystem/8(XMEAS(36)) -> Bus Creator/8  "XMEAS(36)"

== system Simulink_TEP/Process Measurements/Reactor Cooling Outlet Water Temperature ==
  Add : Sum
  Bus Selector1 : BusSelector  OutputSignals=signal4.XMNS(21)
  XMEAS(21) : Outport  PortDimensions=1  VectorParamsAs1DForOutWhenUnconnected=off
  wires:
  [TWR] -> Add/1
  Add/1 -> XMEAS(21)/1  "XMEAS(21)"
  [XMNS] -> Bus Selector1/1
  Bus Selector1/1 -> Add/2  "<XMNS(21)>"

== system Simulink_TEP/Process Measurements/Reactor feed analysis ==
  Bus Creator : BusCreator  Inputs=6
  Bus Selector : BusSelector  OutputSignals=signal1.XST(I;6) = XST(I;7)
  Subsystem : Subsystem
  XMEASR : Outport  VectorParamsAs1DForOutWhenUnconnected=off
  wires:
  [PropertiesStream6] -> Bus Selector/1
  Bus Creator/1 -> XMEASR/1
  Bus Selector/1 -> Subsystem/1(<XST(I;6) = XST(I;7)>)  "<XST(I;6) = XST(I;7)>"
  Subsystem/1(XMEAS(23)) -> Bus Creator/1  "XMEAS(23)"
  Subsystem/2(XMEAS(24)) -> Bus Creator/2  "XMEAS(24)"
  Subsystem/3(XMEAS(25)) -> Bus Creator/3  "XMEAS(25)"
  Subsystem/4(XMEAS(26)) -> Bus Creator/4  "XMEAS(26)"
  Subsystem/5(XMEAS(27)) -> Bus Creator/5  "XMEAS(27)"
  Subsystem/6(XMEAS(28)) -> Bus Creator/6  "XMEAS(28)"

== system Simulink_TEP/Process Measurements/Subsystem3 ==
  Bus Creator : BusCreator  Inputs=4
  "Reactor Feed " : Subsystem
  Reactor Level : Subsystem
  Reactor Pressure : Subsystem
  Reactor Temperature : Subsystem
  Reactor : Outport  VectorParamsAs1DForOutWhenUnconnected=off
  wires:
  Reactor Pressure/1("XMEAS(7) ") -> Bus Creator/2
  Reactor Level/1("XMEAS(8) ") -> Bus Creator/3
  Bus Creator/1 -> Reactor/1
  "Reactor Feed "/1("XMEAS(6) ") -> Bus Creator/1
  Reactor Temperature/1("XMEAS(9) ") -> Bus Creator/4

== system Simulink_TEP/Process Measurements/Subsystem4 ==
  Bus Creator3 : BusCreator  Inputs=5
  Purge Rate : Subsystem
  Separator Level : Subsystem
  Separator Pressure : Subsystem
  Separator Temperature : Subsystem
  Separator Underflow : Subsystem
  Separator : Outport  VectorParamsAs1DForOutWhenUnconnected=off
  wires:
  Bus Creator3/1 -> Separator/1
  Purge Rate/1("XMEAS(10) ") -> Bus Creator3/1
  Separator Temperature/1("XMEAS(11) ") -> Bus Creator3/2
  Separator Level/1("XMEAS(12) ") -> Bus Creator3/3
  Separator Pressure/1("XMEAS(13) ") -> Bus Creator3/4
  Separator Underflow/1("XMEAS(14) ") -> Bus Creator3/5

== system Simulink_TEP/Process Measurements/Subsystem5 ==
  Bus Creator4 : BusCreator  Inputs=5
  Stripper Level : Subsystem
  Stripper Pressure : Subsystem
  Stripper Steam Flow : Subsystem
  Stripper Temperature : Subsystem
  Stripper Underflow : Subsystem
  Stripper : Outport  VectorParamsAs1DForOutWhenUnconnected=off
  wires:
  Stripper Level/1("XMEAS(15) ") -> Bus Creator4/1
  Bus Creator4/1 -> Stripper/1
  Stripper Steam Flow/1("XMEAS(19) ") -> Bus Creator4/5
  Stripper Temperature/1("XMEAS(18) ") -> Bus Creator4/4
  Stripper Pressure/1("XMEAS(16) ") -> Bus Creator4/2
  Stripper Underflow/1("XMEAS(17) ") -> Bus Creator4/3

== system Simulink_TEP/Random number generator/Disturbances I=1-9 ==
  G : Inport
  Bus Creator : BusCreator  Inputs=9
  TESUB7(1) : Subsystem
  TESUB7(2) : Subsystem
  TESUB7(3) : Subsystem
  TESUB7(4) : Subsystem
  TESUB7(5) : Subsystem
  TESUB7(6) : Subsystem
  TESUB7(7) : Subsystem
  TESUB7(8) : Subsystem
  TESUB7(9) : Subsystem
  G1 : Outport  VectorParamsAs1DForOutWhenUnconnected=off
  tag scope: TESUB7=global
  wires:
  G/1 -> TESUB7(1)/1(G)
  TESUB7(1)/2(G_NEW) -> TESUB7(2)/1(G)
  TESUB7(2)/2(G_NEW) -> TESUB7(3)/1(G)
  TESUB7(4)/2(G_NEW) -> TESUB7(5)/1(G)
  TESUB7(5)/2(G_NEW) -> TESUB7(6)/1(G)
  TESUB7(6)/2(G_NEW) -> TESUB7(7)/1(G)
  TESUB7(7)/2(G_NEW) -> TESUB7(8)/1(G)
  TESUB7(8)/2(G_NEW) -> TESUB7(9)/1(G)
  TESUB7(9)/2(G_NEW) -> G1/1
  TESUB7(1)/1(TESUB7(1)) -> Bus Creator/1  "TESUB7_1"
  TESUB7(2)/1(TESUB7(2)) -> Bus Creator/2  "TESUB7_2"
  TESUB7(9)/1(TESUB7(9)) -> Bus Creator/9  "TESUB7_9"
  TESUB7(3)/1(TESUB7(3)) -> Bus Creator/3  "TESUB7_3"
  TESUB7(4)/1(TESUB7(4)) -> Bus Creator/4  "TESUB7_4"
  TESUB7(5)/1(TESUB7(5)) -> Bus Creator/5  "TESUB7_5"
  TESUB7(6)/1(TESUB7(6)) -> Bus Creator/6  "TESUB7_6"
  TESUB7(7)/1(TESUB7(7)) -> Bus Creator/7  "TESUB7_7"
  TESUB7(8)/1(TESUB7(8)) -> Bus Creator/8  "TESUB7_8"
  Bus Creator/1 -> [TESUB7]
  TESUB7(3)/2(G_NEW) -> TESUB7(4)/1(G)

== system Simulink_TEP/Random number generator/Disturbances I=10-12 ==
  G2 : Inport
  Bus Creator : BusCreator  Inputs=3
  TESUB7(10) : Subsystem
  TESUB7(11) : Subsystem
  TESUB7(12) : Subsystem
  G3 : Outport  VectorParamsAs1DForOutWhenUnconnected=off
  tag scope: TESUB7_2=global
  wires:
  TESUB7(12)/2(G_NEW) -> G3/1
  TESUB7(11)/2(G_NEW) -> TESUB7(12)/1(G)
  TESUB7(10)/2(G_NEW) -> TESUB7(11)/1(G)
  TESUB7(10)/1(TESUB7(10)) -> Bus Creator/1  "TESUB7_10"
  TESUB7(11)/1(TESUB7(11)) -> Bus Creator/2  "TESUB7_11"
  TESUB7(12)/1(TESUB7(12)) -> Bus Creator/3  "TESUB7_12"
  Bus Creator/1 -> [TESUB7_2]
  G2/1 -> TESUB7(10)/1(G)

== system Simulink_TEP/Random number generator/Process Measurements XMEAS(I) I=1-22 ==
  G2 : Inport
  Clock3 : Clock
  If Action Subsystem3 : Subsystem  TreatAsAtomicUnit=on
  If3 : If  NumInputs=2  IfExpression=u1>0 & u2==1  ShowElse=off
  Subsystem : Subsystem
  G3 : Outport  VectorParamsAs1DForOutWhenUnconnected=off
  tag scope: XMNS=global
  wires:
  Clock3/1 -> If3/1
  If3/1 -> If Action Subsystem3/Action
  G2/1 -> Subsystem/2(G2), If Action Subsystem3/1(G2)
  If Action Subsystem3/2(G3) -> Subsystem/1(In2)
  Subsystem/1(G3) -> G3/1
  [ISD] -> If3/2
  If Action Subsystem3/1(XMNS) -> [XMNS]

== system Simulink_TEP/Random number generator/Process Measurements XMEAS(I) I=23-36 ==
  G3 : Inport
  Gas Analysis Delay : Subsystem
  If Action Subsystem3 : Subsystem  TreatAsAtomicUnit=on
  Subsystem : Subsystem
  G4 : Outport  VectorParamsAs1DForOutWhenUnconnected=off
  tag scope: XMNS2=global
  wires:
  If Action Subsystem3/1(XMNS) -> [XMNS2]
  G3/1 -> Subsystem/2(G3), If Action Subsystem3/1(G3)
  Subsystem/1(G4) -> G4/1
  If Action Subsystem3/2(G4) -> Subsystem/1(In2)
  Gas Analysis Delay/1(IF(TGAS)) -> If Action Subsystem3/Action

== system Simulink_TEP/Random number generator/Process Measurements XMEAS(I) I=37-41 ==
  G4 : Inport
  Gas Analysis Delay : Subsystem
  If Action Subsystem3 : Subsystem  TreatAsAtomicUnit=on
  Subsystem : Subsystem
  G5 : Outport  VectorParamsAs1DForOutWhenUnconnected=off
  tag scope: XMNS3=global
  wires:
  If Action Subsystem3/2(G5) -> Subsystem/1(In2)
  Subsystem/1(G5) -> G5/1
  If Action Subsystem3/1(XMNS) -> [XMNS3]
  G4/1 -> Subsystem/2(G4), If Action Subsystem3/1(G4)
  Gas Analysis Delay/1(IF(TPROD)) -> If Action Subsystem3/Action

== system Simulink_TEP/Reactor/Holdup of Components in Reactor ==
  CRXR : Inport
  Properties of Stream 6 : Inport  Port=2
  Bus Creator : BusCreator  Inputs=8
  Holdup of Liquid Components in Reactor : Subsystem
  Holdup of Vapour Components in Reactor : Subsystem
  Liquid Component Fraction in Reactor lb-mol : Subsystem
  Subsystem : Subsystem
  Subsystem1 : Subsystem
  UTLR Total Liquid Component holdup in Reactor lb-mol : Sum  Inputs=+
  YP(1) : Subsystem
  YP(2) : Subsystem
  YP(3) : Subsystem
  YP(4) : Subsystem
  YP(5) : Subsystem
  YP(6) : Subsystem
  YP(7) : Subsystem
  YP(8) : Subsystem
  UTLR : Outport  VectorParamsAs1DForOutWhenUnconnected=off
  XLR : Outport  Port=2  PortDimensions=8  VectorParamsAs1DForOutWhenUnconnected=off
  UCVR : Outport  Port=3  VectorParamsAs1DForOutWhenUnconnected=off
  wires:
  YP(3)/1(YY(3)) -> Bus Creator/3  "YY(3)"
  YP(5)/1("YY(5) ") -> Bus Creator/5  "YY(5)"
  YP(6)/1("YY(6) ") -> Bus Creator/6  "YY(6)"
  YP(7)/1("YY(7) ") -> Bus Creator/7  "YY(7)"
  YP(8)/1("YY(8) ") -> Bus Creator/8  "YY(8)"
  CRXR/1 -> YP(8)/2(CRXR(8)), YP(7)/2(CRXR(7)), YP(6)/2(CRXR(6)), YP(5)/2(CRXR(5)), YP(4)/2(CRXR(4)), YP(3)/2(CRXR(3)), YP(1)/2(CRXR(1))
  UTLR Total Liquid Component holdup in Reactor lb-mol/1 -> Liquid Component Fraction in Reactor lb-mol/1(UTLR), UTLR/1
  Holdup of Liquid Components in Reactor/1(UCLR) -> UTLR Total Liquid Component holdup in Reactor lb-mol/1, Liquid Component Fraction in Reactor lb-mol/2(UCLR)
  YP(2)/1(YY(2)) -> Bus Creator/2  "YY(2)"
  YP(1)/1(YY(1)) -> Bus Creator/1  "YY(1)"
  YP(4)/1("YY(4) ") -> Bus Creator/4  "YY(4)"
  Holdup of Vapour Components in Reactor/1(UCVR) -> UCVR/1
  Liquid Component Fraction in Reactor lb-mol/1(XLR) -> XLR/1
  Bus Creator/1 -> Holdup of Vapour Components in Reactor/1(YY(1:8)), Holdup of Liquid Components in Reactor/1(YY(1:8))
  Properties of Stream 6/1 -> Subsystem/1(Properties of Stream 6)
  Subsystem1/1(FCM(I;8)) -> YP(8)/3(FCM(8,8)), YP(7)/3(FCM(7,8)), YP(6)/3(FCM(6,8)), YP(5)/3(FCM(5,8)), YP(4)/3(FCM(4,8)), YP(3)/3(FCM(3,8)), YP(2)/2(FCM(2,8)), YP(1)/3(FCM(1,8))
  Subsystem/1(FCM(I;7)) -> YP(1)/1(FCM(1,7)), YP(8)/1(FCM(8,7)), YP(7)/1(FCM(7,7)), YP(6)/1(FCM(6,7)), YP(5)/1(FCM(5,7)), YP(4)/1(FCM(4,7)), YP(3)/1(FCM(3,7)), YP(2)/1(FCM(2,7))

== system Simulink_TEP/Reactor/Internal energy of reactor ==
  RH : Inport
  QUR : Inport  Port=2
  Properties of Stream 6 : Inport  Port=3
  Add : Sum  Inputs=3
  Bus Selector : BusSelector  OutputSignals=HST(6) = HST(7),FTM(6) = FTM(7)
  Bus Selector1 : BusSelector  OutputSignals=signal1.HST(8),signal1.FTM(8)
  Product : Product
  Product1 : Product
  Subtract : Sum  Inputs=+-
  YP(9) : Integrator  InitialConditionSource=external
  YY(9) : Constant  Value=2.808522723
  "YY(9) " : Outport  VectorParamsAs1DForOutWhenUnconnected=off
  wires:
  Bus Selector/1 -> Product/1  "<HST(6) = HST(7)>"
  Bus Selector/2 -> Product/2  "<FTM(6) = FTM(7)>"
  Bus Selector1/2 -> Product1/2  "<FTM(8)>"
  Bus Selector1/1 -> Product1/1  "<HST(8)>"
  Product/1 -> Subtract/1
  Product1/1 -> Subtract/2
  Subtract/1 -> Add/1
  RH/1 -> Add/2
  QUR/1 -> Add/3
  YP(9)/1 -> "YY(9) "/1
  YY(9)/1 -> YP(9)/2
  Add/1 -> YP(9)/1
  Properties of Stream 6/1 -> Bus Selector/1
  [PropertiesStream8] -> Bus Selector1/1

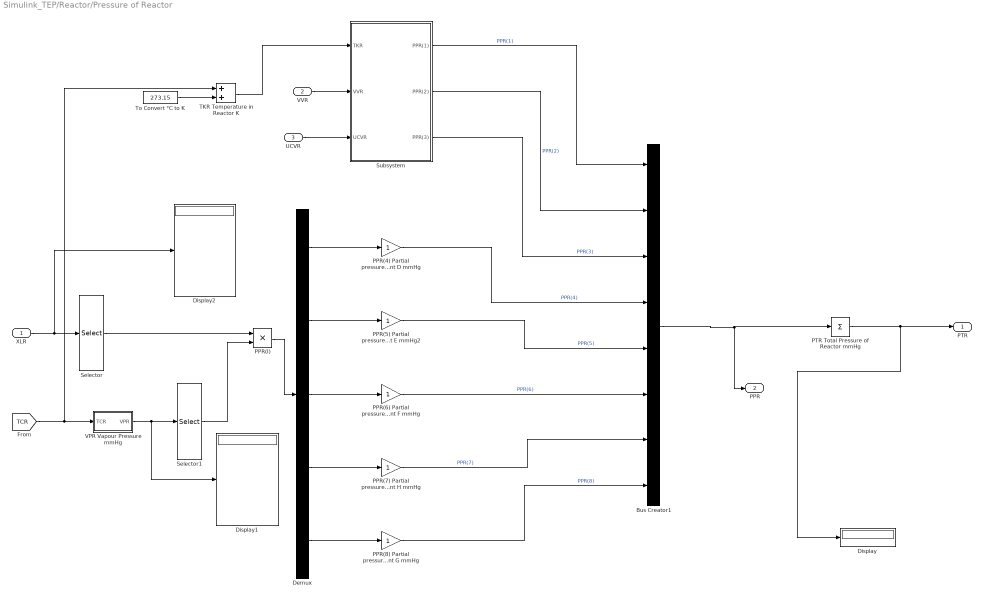
== system Simulink_TEP/Reactor/Pressure of Reactor ==
  XLR : Inport
  VVR : Inport  Port=2
  UCVR : Inport  Port=3
  Bus Creator1 : BusCreator  Inputs=8
  Demux : Demux  Outputs=5
  Display : Display
  Display1 : Display
  Display2 : Display
  PPR(4) Partial pressure of Component D mmHg : Gain
  PPR(5) Partial pressure of Component E mmHg2 : Gain
  PPR(6) Partial pressure of Component F mmHg : Gain
  PPR(7) Partial pressure of Component H mmHg : Gain
  PPR(8) Partial pressure of Component G mmHg : Gain
  PPR(I) : Product
  PTR Total Pressure of Reactor mmHg : Sum  Inputs=+
  Selector : Selector  InputPortWidth=8  IndexOptions=Index vector (dialog)  Indices=[4 5 6 7 8]  OutputSizes=1
  Selector1 : Selector  InputPortWidth=8  IndexOptions=Index vector (dialog)  Indices=[4 5 6 7 8]  OutputSizes=1
  Subsystem : Subsystem
  TKR Temperature in Reactor K : Sum
  To Convert °C to K : Constant  Value=273.15
  VPR Vapour Pressure mmHg : Subsystem
  PTR : Outport  PortDimensions=1  VectorParamsAs1DForOutWhenUnconnected=off
  PPR : Outport  Port=2  PortDimensions=8  VectorParamsAs1DForOutWhenUnconnected=off
  wires:
  PPR(7) Partial pressure of Component H mmHg/1 -> Bus Creator1/7  "PPR(7)"
  VPR Vapour Pressure mmHg/1(VPR) -> Display1/1, Selector1/1
  PPR(I)/1 -> Demux/1
  Demux/2 -> PPR(5) Partial pressure of Component E mmHg2/1
  XLR/1 -> Display2/1, Selector/1
  PTR Total Pressure of Reactor mmHg/1 -> Display/1, PTR/1
  PPR(8) Partial pressure of Component G mmHg/1 -> Bus Creator1/8  "PPR(8)"
  PPR(6) Partial pressure of Component F mmHg/1 -> Bus Creator1/6  "PPR(6)"
  Demux/5 -> PPR(8) Partial pressure of Component G mmHg/1
  Selector/1 -> PPR(I)/1
  UCVR/1 -> Subsystem/3(UCVR)
  Selector1/1 -> PPR(I)/2
  PPR(4) Partial pressure of Component D mmHg/1 -> Bus Creator1/4  "PPR(4)"
  PPR(5) Partial pressure of Component E mmHg2/1 -> Bus Creator1/5  "PPR(5)"
  Demux/1 -> PPR(4) Partial pressure of Component D mmHg/1
  Subsystem/3(PPR(3)) -> Bus Creator1/3  "PPR(3)"
  Demux/3 -> PPR(6) Partial pressure of Component F mmHg/1
  Demux/4 -> PPR(7) Partial pressure of Component H mmHg/1
  Bus Creator1/1 -> PPR/1, PTR Total Pressure of Reactor mmHg/1
  Subsystem/2(PPR(2)) -> Bus Creator1/2  "PPR(2)"
  Subsystem/1(PPR(1)) -> Bus Creator1/1  "PPR(1)"
  [TCR] -> TKR Temperature in Reactor K/1, VPR Vapour Pressure mmHg/1(TCR)
  TKR Temperature in Reactor K/1 -> Subsystem/1(TKR)
  VVR/1 -> Subsystem/2(VVR)
  To Convert °C to K/1 -> TKR Temperature in Reactor K/2

== system Simulink_TEP/Reactor/Reaction Rates ==
  VVR : Inport
  PPR : Inport  Port=2
  Component reaction rate lb-mol/h : Subsystem
  Reaction Heat MBtu/h : Subsystem
  Reaction rates lb-mol/h : Subsystem
  TKR Temperature in Reactor K : Sum
  To Convert °C to K : Constant  Value=273.15
  "RH " : Outport  VectorParamsAs1DForOutWhenUnconnected=off
  CRXR : Outport  Port=2  PortDimensions=7  VectorParamsAs1DForOutWhenUnconnected=off
  wires:
  PPR/1 -> Reaction rates lb-mol/h/2(PPR)
  TKR Temperature in Reactor K/1 -> Reaction rates lb-mol/h/1(TKR)
  To Convert °C to K/1 -> TKR Temperature in Reactor K/1
  [TCR] -> TKR Temperature in Reactor K/2
  Component reaction rate lb-mol/h/1(CRXR) -> CRXR/1
  Reaction rates lb-mol/h/1(RR) -> Reaction Heat MBtu/h/1(RR), Component reaction rate lb-mol/h/1(RR)
  VVR/1 -> Reaction rates lb-mol/h/3(VVR)
  Reaction Heat MBtu/h/1(RH) -> "RH "/1

== system Simulink_TEP/Reactor/Reactor Heat exchanger ==
  Position of Valve 10 % : Subsystem
  Position of Valve 12 % : Subsystem
  Reactor Heat exchanger : Subsystem
  "VRNG(10) Max flow of water through valve " : Constant  Value=1000
  QUR : Outport  VectorParamsAs1DForOutWhenUnconnected=off
  wires:
  "VRNG(10) Max flow of water through valve "/1 -> Reactor Heat exchanger/3(VRNG(10))
  [VLR] -> Reactor Heat exchanger/1(VLR)
  Position of Valve 12 %/1("YY(50) ") -> Reactor Heat exchanger/4(VPOS(12))
  Position of Valve 10 %/1("YY(48) ") -> Reactor Heat exchanger/2(VPOS(10))
  [TCR] -> Reactor Heat exchanger/5(TCR)
  Reactor Heat exchanger/1("QUR ") -> QUR/1

== system Simulink_TEP/Reactor/Stream 8 ==
  TST(8) : Inport
  XTS(I,8) : Inport  Port=2
  Bus Creator : BusCreator  Inputs=6
  FCM(I,8) Component molar flow of Stream 8 lb-mol/h : Product
  FTM(8) : Product  Inputs=*/
  HST(8) Molar Enthalpy of Stream 8 MBtu/lb-mol : Subsystem
  ITY : Constant
  Subsystem : Subsystem
  XMWS(8) Molecular weight of Stream 8 lb/lb-mol : Subsystem
  Properties of Stream 8 : Outport  VectorParamsAs1DForOutWhenUnconnected=off
  wires:
  ITY/1 -> Bus Creator/6, HST(8) Molar Enthalpy of Stream 8 MBtu/lb-mol/1(ITY)  "Phase"
  XTS(I,8)/1 -> XMWS(8) Molecular weight of Stream 8 lb/lb-mol/1(XST(I,8)), FCM(I,8) Component molar flow of Stream 8 lb-mol/h/2, Bus Creator/1, HST(8) Molar Enthalpy of Stream 8 MBtu/lb-mol/3(XST(I,I))  "XST(I;8)"
  TST(8)/1 -> Bus Creator/2, HST(8) Molar Enthalpy of Stream 8 MBtu/lb-mol/2(T)  "TST(8)"
  HST(8) Molar Enthalpy of Stream 8 MBtu/lb-mol/1("H ") -> Bus Creator/3  "HST(8)"
  XMWS(8) Molecular weight of Stream 8 lb/lb-mol/1(XMWS(8)) -> FTM(8)/2
  FTM(8)/1 -> FCM(I,8) Component molar flow of Stream 8 lb-mol/h/1, Bus Creator/4  "FTM(8)"
  FCM(I,8) Component molar flow of Stream 8 lb-mol/h/1 -> Bus Creator/5  "FCM(I;8)"
  Bus Creator/1 -> Properties of Stream 8/1
  Subsystem/1("FLMS ") -> FTM(8)/1

== system Simulink_TEP/Reactor/TCR Initial Temperature in Reactor °C  ==
  UTLR : Inport
  ETR : Inport  Port=2  PortDimensions=1
  XLR : Inport  Port=3  PortDimensions=8
  "AG(I) Coefficient A to determine Enthalpy MBtu/lb·°F " : Constant  Value=AG
  "AH(I) Coefficient A to determine Enthalpy MBtu/lb·°F " : Constant  Value=AH
  AV(I) Coefficient AV to determine Enthalpy MBtu/lb : Constant  Value=AV
  BG(I) Coefficient B to determine Enthalpy MBtu/lb·°F² : Constant  Value=BG
  BH(I) Coefficient B to determine Enthalpy MBtu/lb·°F² : Constant  Value=BH
  CG(I) Coefficient C to determine Enthalpy MBtu/lb·°F³ : Constant  Value=CG
  CH(I) Coefficient C to determine Enthalpy MBtu/lb·°F³ : Constant  Value=CH
  Delay : Delay  DelayLength=1  InitialCondition=0
  Display1 : Display
  Display4 : Display
  IC : InitialCondition  Value=0
  ITY : Constant  Value=0
  MATLAB Function : MATLAB Function  TreatAsAtomicUnit=on
  "XMW(I) Molecular weight of components lb/lb-mol " : Constant  Value=XMW
  TCR : Outport  PortDimensions=1  VectorParamsAs1DForOutWhenUnconnected=off
  wires:
  MATLAB Function/1(TCR) -> Delay/1, TCR/1, Display4/1
  IC/1 -> MATLAB Function/13("TCR ")
  "AG(I) Coefficient A to determine Enthalpy MBtu/lb·°F "/1 -> MATLAB Function/4(AG)
  AV(I) Coefficient AV to determine Enthalpy MBtu/lb/1 -> MATLAB Function/7(AV)
  MATLAB Function/2(J) -> Display1/1
  ETR/1 -> MATLAB Function/10(ETR)
  CH(I) Coefficient C to determine Enthalpy MBtu/lb·°F³/1 -> MATLAB Function/3(CH)
  UTLR/1 -> MATLAB Function/11(UTLR)
  ITY/1 -> MATLAB Function/12(ITY)
  "XMW(I) Molecular weight of components lb/lb-mol "/1 -> MATLAB Function/8(XMW)
  XLR/1 -> MATLAB Function/9(XLR)
  "AH(I) Coefficient A to determine Enthalpy MBtu/lb·°F "/1 -> MATLAB Function/1(AH)
  CG(I) Coefficient C to determine Enthalpy MBtu/lb·°F³/1 -> MATLAB Function/6(CG)
  BH(I) Coefficient B to determine Enthalpy MBtu/lb·°F²/1 -> MATLAB Function/2(BH)
  BG(I) Coefficient B to determine Enthalpy MBtu/lb·°F²/1 -> MATLAB Function/5(BG)
  Delay/1 -> IC/1

== system Simulink_TEP/Reactor/Total Vapour Component Holdup in Reactor ==
  VVR : Inport
  XVR : Inport  Port=2
  Display9 : Display
  RG Universal Gas Constant ft³·mmHg/K·lb-mol : Constant  Value=998.9
  TKR Temperature in Reactor K : Sum
  To Convert °C to K : Constant  Value=273.15
  UCVR(I) Vapour Component Holdup in Reactor lb-mol2 : Product  Inputs=**
  UTVR Total Vapour Component Holdup in Reactor lb-mol : Product  Inputs=**//
  wires:
  RG Universal Gas Constant ft³·mmHg/K·lb-mol/1 -> UTVR Total Vapour Component Holdup in Reactor lb-mol/3
  VVR/1 -> UTVR Total Vapour Component Holdup in Reactor lb-mol/2
  [PTR] -> UTVR Total Vapour Component Holdup in Reactor lb-mol/1
  UTVR Total Vapour Component Holdup in Reactor lb-mol/1 -> UCVR(I) Vapour Component Holdup in Reactor lb-mol2/1
  TKR Temperature in Reactor K/1 -> UTVR Total Vapour Component Holdup in Reactor lb-mol/4
  To Convert °C to K/1 -> TKR Temperature in Reactor K/2
  [TCR] -> TKR Temperature in Reactor K/1
  UCVR(I) Vapour Component Holdup in Reactor lb-mol2/1 -> Display9/1
  XVR/1 -> UCVR(I) Vapour Component Holdup in Reactor lb-mol2/2

== system Simulink_TEP/Reactor/Vapour Component Fraction in Reactor ==
  PPR : Inport
  Bus Creator2 : BusCreator  Inputs=8
  Bus Selector1 : BusSelector  OutputSignals=PPR(1),PPR(2),PPR(3),PPR(4),PPR(5),PPR(6),PPR(7),PPR(8)
  XVR(1) : Product  Inputs=*/
  XVR(2) : Product  Inputs=*/
  XVR(3) : Product  Inputs=*/
  XVR(4) : Product  Inputs=*/
  XVR(5) : Product  Inputs=*/
  XVR(6) : Product  Inputs=*/
  XVR(7) : Product  Inputs=*/
  XVR(8) : Product  Inputs=*/
  XVR : Outport  PortDimensions=8  VectorParamsAs1DForOutWhenUnconnected=off
  wires:
  XVR(5)/1 -> Bus Creator2/5
  XVR(8)/1 -> Bus Creator2/8
  Bus Selector1/3 -> XVR(3)/1  "<PPR(3)>"
  XVR(4)/1 -> Bus Creator2/4
  Bus Selector1/7 -> XVR(7)/1  "<PPR(7)>"
  Bus Selector1/6 -> XVR(6)/1  "<PPR(6)>"
  XVR(7)/1 -> Bus Creator2/7
  Bus Selector1/2 -> XVR(2)/1  "<PPR(2)>"
  XVR(3)/1 -> Bus Creator2/3
  XVR(6)/1 -> Bus Creator2/6
  PPR/1 -> Bus Selector1/1
  XVR(2)/1 -> Bus Creator2/2
  Bus Selector1/1 -> XVR(1)/1  "<PPR(1)>"
  Bus Selector1/8 -> XVR(8)/1  "<PPR(8)>"
  Bus Creator2/1 -> XVR/1
  XVR(1)/1 -> Bus Creator2/1
  Bus Selector1/5 -> XVR(5)/1  "<PPR(5)>"
  Bus Selector1/4 -> XVR(4)/1  "<PPR(4)>"
  [PTR] -> XVR(8)/2, XVR(7)/2, XVR(6)/2, XVR(5)/2, XVR(4)/2, XVR(3)/2, XVR(2)/2, XVR(1)/2
